simulink model "MODEL_FULL_SYSTEM_MUTUAL"  (Simulink 7.8)
settings: Solver=ode1  StartTime=0.0  StopTime=inf  FixedStep=Ts  MaxStep=1e-3  RelTol=1e-3
PostLoadFcn:
  | Ts=80e-6; relays_settings_init;
InitFcn:
  | Ts=80e-6; relays_settings_init;
values from neighbouring files (symbols this model uses):
  relay_sets = xlsread('relay_settings_10272015.xlsx')    [relays_settings_init.m]
undefined symbols (not defined in the file or in its folder): dfilt, DiscIntNeverNeededParam, fdesignblkfcn, gcbh, Left, opmodbus_cb, ph, Right, type, V, X
libraries: simulink x72, modbus_lib x40, cables_lib x36, rtio_opalrt_common x21, rtlab x20, transformer_lib x13, dynamic_load_lib x12, powerlib x6, simulink_extras x6, ssn_lib x5, discretizing x4, rteventslib x4
(part 5 of 7)

== system MODEL_FULL_SYSTEM_MUTUAL/SS_Slave/Input to UDP Block - v1 ==
  note: Using phase A:
      | 1)  voltage 1MVA gen
      | 2) voltage 4MVA gen
      | 3) battery current
  note: gens are operating at higher voltage than 1pu - instead of mult by 1.414, I mult by 1.214
  ms : Inport
  batt : Inport  Port=2
  gen : Inport  Port=3
  Bus Selector1 : BusSelector  OutputSignals=SEL_787_Relay1.m.P,SEL_787_Relay2.m.P,SEL_787_Relay3.m.P,SEL_787_Relay4.m.P,SEL_787_Relay5.m.P,SEL_787_Relay6.m.P,SEL_787_Relay7.m.P,SEL_787_Relay8.m.P,SEL_787_Relay9.m.P,SEL_787_Relay10.m.P,SEL_787_Relay11.m.P,SEL_787_Relay12.m.P,SEL_787_Relay13.m.P,SEL_787_Relay14.m.P,SEL_787_Relay15.m.P,SEL_787_Relay16.m.P,SEL_787_Relay17.m.P,SEL_787_Relay18.m.P,SEL_787_Relay19.m.P
  Bus Selector2 : BusSelector  OutputSignals=SEL_787_Relay1.m.Q,SEL_787_Relay2.m.Q,SEL_787_Relay3.m.Q,SEL_787_Relay4.m.Q,SEL_787_Relay5.m.Q,SEL_787_Relay6.m.Q,SEL_787_Relay7.m.Q,SEL_787_Relay8.m.Q,SEL_787_Relay9.m.Q,SEL_787_Relay10.m.Q,SEL_787_Relay11.m.Q,SEL_787_Relay12.m.Q,SEL_787_Relay13.m.Q,SEL_787_Relay14.m.Q,SEL_787_Relay15.m.Q,SEL_787_Relay16.m.Q,SEL_787_Relay17.m.Q,SEL_787_Relay18.m.Q,SEL_787_Relay19.m.Q
  Bus Selector3 : BusSelector  OutputSignals=SEL_787_Relay1.m.Vpu,SEL_787_Relay2.m.Vpu,SEL_787_Relay3.m.Vpu,SEL_787_Relay4.m.Vpu,SEL_787_Relay5.m.Vpu,SEL_787_Relay6.m.Vpu,SEL_787_Relay7.m.Vpu,SEL_787_Relay8.m.Vpu,SEL_787_Relay9.m.Vpu,SEL_787_Relay10.m.Vpu,SEL_787_Relay11.m.Vpu,SEL_787_Relay12.m.Vpu,SEL_787_Relay13.m.Vpu,SEL_787_Relay14.m.Vpu,SEL_787_Relay15.m.Vpu,SEL_787_Relay16.m.Vpu,SEL_787_Relay17.m.Vpu,SEL_787_Relay18.m.Vpu,SEL_787_Relay19.m.Vpu
  Bus Selector4 : BusSelector  OutputSignals=SEL_787_Relay1.m.freq,SEL_787_Relay2.m.freq,SEL_787_Relay3.m.freq,SEL_787_Relay4.m.freq,SEL_787_Relay5.m.freq,SEL_787_Relay6.m.freq,SEL_787_Relay7.m.freq,SEL_787_Relay8.m.freq,SEL_787_Relay9.m.freq,SEL_787_Relay10.m.freq,SEL_787_Relay11.m.freq,SEL_787_Relay12.m.freq,SEL_787_Relay13.m.freq,SEL_787_Relay14.m.freq,SEL_787_Relay15.m.freq,SEL_787_Relay16.m.freq,SEL_787_Relay17.m.freq,SEL_787_Relay18.m.freq,SEL_787_Relay19.m.freq
  Bus Selector5 : BusSelector  OutputSignals=SEL_787_Relay1.m.status,SEL_787_Relay2.m.status,SEL_787_Relay3.m.status,SEL_787_Relay4.m.status,SEL_787_Relay5.m.status,SEL_787_Relay6.m.status,SEL_787_Relay7.m.status,SEL_787_Relay8.m.status,SEL_787_Relay9.m.status,SEL_787_Relay10.m.status,SEL_787_Relay11.m.status,SEL_787_Relay12.m.status,SEL_787_Relay13.m.status,SEL_787_Relay14.m.status,SEL_787_Relay15.m.status,SEL_787_Relay16.m.status,SEL_787_Relay17.m.status,SEL_787_Relay18.m.status,SEL_787_Relay19.m.status
  Bus Selector6 : BusSelector  OutputSignals=Capacity.Capacity (signal 2)
  Bus Selector7 : BusSelector  OutputSignals=SEL_787_Relay1.m.pf
  Bus Selector8 : BusSelector  OutputSignals=gal_per_hr_1MVA,gal_per_hr_4MVA
  Bus Selector9 : BusSelector  OutputSignals=SEL_787_Relay7.m.Vabc,SEL_787_Relay8.m.Vabc,SEL_787_Relay13.m.Iabc
  Data Type Conversion : DataTypeConversion
  Demux : Demux  Outputs=3
  Demux1 : Demux  Outputs=3
  Demux2 : Demux  Outputs=3
  Gain : Gain  Gain=1.214/460
  Gain1 : Gain  Gain=1.214/13800
  Gain2 : Gain  Gain=1/1000
  Gain3 : Gain  Gain=1/1000
  Gain4 : Gain  Gain=1/(4E6/(1.732*2047))
  Mux : Mux  Inputs=3
  Mux{1..5} (5 alike) : Mux  Inputs=20
  Mux6 : Mux  Inputs=2
  waveforms : Outport
  kW : Outport  Port=2
  kvar : Outport  Port=3
  Vpu : Outport  Port=4
  freq : Outport  Port=5
  breaker_status : Outport  Port=6
  Batt SoC : Outport  Port=7
  PF at PCC : Outport  Port=8
  gen_fuel : Outport  Port=9
  wires:
  Bus Selector4/19 -> Mux4/19  "<freq>"
  Bus Selector4/18 -> Mux4/18  "<freq>"
  Bus Selector4/17 -> Mux4/17  "<freq>"
  Bus Selector4/16 -> Mux4/16  "<freq>"
  Bus Selector4/15 -> Mux4/15  "<freq>"
  Bus Selector4/14 -> Mux4/14  "<freq>"
  Bus Selector4/13 -> Mux4/13  "<freq>"
  Bus Selector4/12 -> Mux4/12  "<freq>"
  Bus Selector4/11 -> Mux4/11  "<freq>"
  Bus Selector4/10 -> Mux4/10  "<freq>"
  Bus Selector4/9 -> Mux4/9  "<freq>"
  Bus Selector4/8 -> Mux4/8  "<freq>"
  Bus Selector4/7 -> Mux4/7  "<freq>"
  Bus Selector4/6 -> Mux4/6  "<freq>"
  Bus Selector4/5 -> Mux4/5  "<freq>"
  Bus Selector4/4 -> Mux4/4  "<freq>"
  Bus Selector4/3 -> Mux4/3  "<freq>"
  Bus Selector4/2 -> Mux4/2  "<freq>"
  Bus Selector4/1 -> Mux4/1  "<freq>"
  Gain4/1 -> Demux2/1
  Data Type Conversion/1 -> breaker_status/1
  Bus Selector9/1 -> Gain/1  "<Vabc>"
  Bus Selector9/3 -> Gain4/1  "<Iabc>"
  Bus Selector9/2 -> Gain1/1  "<Vabc>"
  Demux1/1 -> Mux/2
  Demux/1 -> Mux/1
  Demux2/1 -> Mux/3
  Gain/1 -> Demux/1
  Gain1/1 -> Demux1/1
  ms/1 -> Bus Selector9/1, Bus Selector1/1, Bus Selector2/1, Bus Selector3/1, Bus Selector4/1, Bus Selector5/1, Bus Selector7/1
  Mux/1 -> waveforms/1
  Bus Selector1/1 -> Mux1/1  "<P>"
  Bus Selector1/2 -> Mux1/2  "<P>"
  Bus Selector1/3 -> Mux1/3  "<P>"
  Bus Selector1/4 -> Mux1/4  "<P>"
  Bus Selector1/5 -> Mux1/5  "<P>"
  Bus Selector1/6 -> Mux1/6  "<P>"
  Bus Selector1/7 -> Mux1/7  "<P>"
  Bus Selector1/8 -> Mux1/8  "<P>"
  Bus Selector1/9 -> Mux1/9  "<P>"
  Bus Selector1/10 -> Mux1/10  "<P>"
  Bus Selector1/11 -> Mux1/11  "<P>"
  Bus Selector1/12 -> Mux1/12  "<P>"
  Bus Selector1/13 -> Mux1/13  "<P>"
  Bus Selector1/14 -> Mux1/14  "<P>"
  Bus Selector1/15 -> Mux1/15  "<P>"
  Bus Selector1/16 -> Mux1/16  "<P>"
  Bus Selector1/17 -> Mux1/17  "<P>"
  Bus Selector1/18 -> Mux1/18  "<P>"
  Bus Selector1/19 -> Mux1/19  "<P>"
  Mux1/1 -> Gain2/1
  Gain2/1 -> kW/1
  Bus Selector2/1 -> Mux2/1  "<Q>"
  Bus Selector2/2 -> Mux2/2  "<Q>"
  Bus Selector2/3 -> Mux2/3  "<Q>"
  Bus Selector2/4 -> Mux2/4  "<Q>"
  Bus Selector2/5 -> Mux2/5  "<Q>"
  Bus Selector2/6 -> Mux2/6  "<Q>"
  Bus Selector2/7 -> Mux2/7  "<Q>"
  Bus Selector2/8 -> Mux2/8  "<Q>"
  Bus Selector2/9 -> Mux2/9  "<Q>"
  Bus Selector2/10 -> Mux2/10  "<Q>"
  Bus Selector2/11 -> Mux2/11  "<Q>"
  Bus Selector2/12 -> Mux2/12  "<Q>"
  Bus Selector2/13 -> Mux2/13  "<Q>"
  Bus Selector2/14 -> Mux2/14  "<Q>"
  Bus Selector2/15 -> Mux2/15  "<Q>"
  Bus Selector2/16 -> Mux2/16  "<Q>"
  Bus Selector2/17 -> Mux2/17  "<Q>"
  Bus Selector2/18 -> Mux2/18  "<Q>"
  Bus Selector2/19 -> Mux2/19  "<Q>"
  Mux2/1 -> Gain3/1
  Gain3/1 -> kvar/1
  Bus Selector3/1 -> Mux3/1  "<Vpu>"
  Bus Selector3/2 -> Mux3/2  "<Vpu>"
  Bus Selector3/3 -> Mux3/3  "<Vpu>"
  Bus Selector3/4 -> Mux3/4  "<Vpu>"
  Bus Selector3/5 -> Mux3/5  "<Vpu>"
  Bus Selector3/6 -> Mux3/6  "<Vpu>"
  Bus Selector3/7 -> Mux3/7  "<Vpu>"
  Bus Selector3/8 -> Mux3/8  "<Vpu>"
  Bus Selector3/9 -> Mux3/9  "<Vpu>"
  Bus Selector3/10 -> Mux3/10  "<Vpu>"
  Bus Selector3/11 -> Mux3/11  "<Vpu>"
  Bus Selector3/12 -> Mux3/12  "<Vpu>"
  Bus Selector3/13 -> Mux3/13  "<Vpu>"
  Bus Selector3/14 -> Mux3/14  "<Vpu>"
  Bus Selector3/15 -> Mux3/15  "<Vpu>"
  Bus Selector3/16 -> Mux3/16  "<Vpu>"
  Bus Selector3/17 -> Mux3/17  "<Vpu>"
  Bus Selector3/18 -> Mux3/18  "<Vpu>"
  Bus Selector3/19 -> Mux3/19  "<Vpu>"
  Mux3/1 -> Vpu/1
  Mux4/1 -> freq/1
  Mux5/1 -> Data Type Conversion/1
  batt/1 -> Bus Selector6/1
  Bus Selector6/1 -> Batt SoC/1  "<Capacity (signal 2)>"
  Bus Selector7/1 -> PF at PCC/1  "<pf>"
  Bus Selector5/1 -> Mux5/1  "<status>"
  Bus Selector5/2 -> Mux5/2  "<status>"
  Bus Selector5/3 -> Mux5/3  "<status>"
  Bus Selector5/4 -> Mux5/4  "<status>"
  Bus Selector5/5 -> Mux5/5  "<status>"
  Bus Selector5/6 -> Mux5/6  "<status>"
  Bus Selector5/7 -> Mux5/7  "<status>"
  Bus Selector5/8 -> Mux5/8  "<status>"
  Bus Selector5/9 -> Mux5/9  "<status>"
  Bus Selector5/10 -> Mux5/10  "<status>"
  Bus Selector5/11 -> Mux5/11  "<status>"
  Bus Selector5/12 -> Mux5/12  "<status>"
  Bus Selector5/13 -> Mux5/13  "<status>"
  Bus Selector5/14 -> Mux5/14  "<status>"
  Bus Selector5/15 -> Mux5/15  "<status>"
  Bus Selector5/16 -> Mux5/16  "<status>"
  Bus Selector5/17 -> Mux5/17  "<status>"
  Bus Selector5/18 -> Mux5/18  "<status>"
  Bus Selector5/19 -> Mux5/19  "<status>"
  gen/1 -> Bus Selector8/1
  Bus Selector8/1 -> Mux6/1  "<gal_per_hr_1MVA>"
  Bus Selector8/2 -> Mux6/2  "<gal_per_hr_4MVA>"
  Mux6/1 -> gen_fuel/1

== system MODEL_FULL_SYSTEM_MUTUAL/SS_Slave/Number of seconds of recording ==
  Compare To Constant1 : simulink/Logic and Bit Operations/Compare To Constant  relop=>=  const=time_s  OutDataTypeStr=boolean
  Increment : Subsystem
  Integrator : Integrator  ExternalReset=rising
  Memory : Memory
  Slope : Constant
  file suffix : Outport
  wires:
  Slope/1 -> Integrator/1
  Integrator/1 -> Compare To Constant1/1
  Compare To Constant1/1 -> Memory/1, Increment/Trigger  "limit reached"
  Memory/1 -> Integrator/2
  Increment/1(Out1) -> file suffix/1

== system MODEL_FULL_SYSTEM_MUTUAL/SS_Slave/Trigg_machine ==
  Write : Inport
  Odd : Inport  Port=2
  Even : Inport  Port=3
  Bitwise Operator : simulink/Logic and Bit Operations/Bitwise Operator  logicop=AND  UseBitMask=off  NumInputPorts=2  BitMask=bin2dec('11011001')  BitMaskRealWorld=Stored Integer
  Bitwise Operator1 : simulink/Logic and Bit Operations/Bitwise Operator  logicop=AND  UseBitMask=off  NumInputPorts=2  BitMask=bin2dec('11011001')  BitMaskRealWorld=Stored Integer
  Data Type Conversion : DataTypeConversion
  Data Type Conversion1 : DataTypeConversion
  Double2uint8 : DataTypeConversion
  Trig_odd : Outport
  Trig_even : Outport  Port=2
  wires:
  Double2uint8/1 -> Bitwise Operator1/1, Bitwise Operator/2
  Write/1 -> Double2uint8/1
  Odd/1 -> Bitwise Operator/1
  Data Type Conversion1/1 -> Trig_even/1
  Data Type Conversion/1 -> Trig_odd/1
  Even/1 -> Bitwise Operator1/2
  Bitwise Operator1/1 -> Data Type Conversion1/1
  Bitwise Operator/1 -> Data Type Conversion/1

== system MODEL_FULL_SYSTEM_MUTUAL/SS_Slave/isOddOrEven ==
  note: Si cette différence est égale à 0, c'est que le
      | nombre en entrée est pair, sinon c'est qu'il est impair.
  note: Effectuer la différence entre le nombre en entrée,
      | et sa moitié arrondie multipliée par 2.
  Index : Inport
  Compare To Zero : simulink/Logic and Bit Operations/Compare To Zero  relop=~=  OutDataTypeStr=boolean  ZeroCross=off
  Compare To Zero1 : simulink/Logic and Bit Operations/Compare To Zero  relop===  OutDataTypeStr=boolean  ZeroCross=off
  Constant3 : Constant  Value=2
  Divide : Product  Inputs=*/  OutDataTypeStr=double
  Produit : Product  Inputs=**  OutDataTypeStr=double
  Rounding Function : Rounding
  Sum : Sum  Inputs=|+-
  isOdd : Outport
  isEven : Outport  Port=2
  wires:
  Compare To Zero1/1 -> isEven/1
  Compare To Zero/1 -> isOdd/1
  Sum/1 -> Compare To Zero1/1, Compare To Zero/1
  Produit/1 -> Sum/2
  Rounding Function/1 -> Produit/1
  Index/1 -> Sum/1, Divide/1
  Divide/1 -> Rounding Function/1
  Constant3/1 -> Produit/2, Divide/2

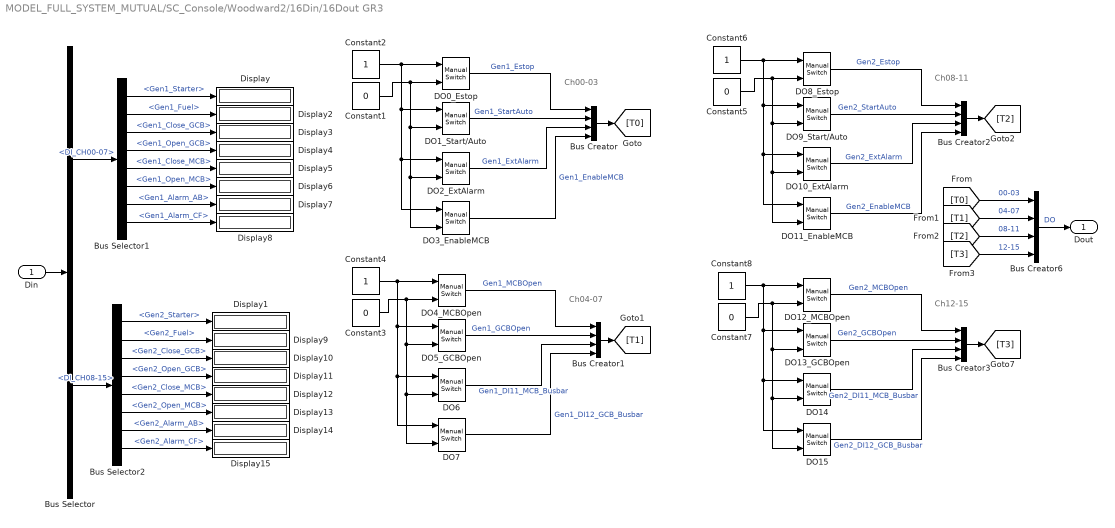
== system MODEL_FULL_SYSTEM_MUTUAL/SC_Console/Woodward2/16Din/16Dout GR3 ==
  note: Ch00-03
  note: Ch04-07
  note: Ch08-11
  note: Ch12-15
  Din : Inport
  Bus Creator{,1..3,6} (5 alike) : BusCreator
  Bus Selector : BusSelector  OutputSignals=DIN.DI_CH00-07,DIN.DI_CH08-15
  Bus Selector1 : BusSelector  OutputSignals=Gen1_Starter,Gen1_Fuel,Gen1_Close_GCB,Gen1_Open_GCB,Gen1_Close_MCB,Gen1_Open_MCB,Gen1_Alarm_AB,Gen1_Alarm_CF
  Bus Selector2 : BusSelector  OutputSignals=Gen2_Starter,Gen2_Fuel,Gen2_Close_GCB,Gen2_Open_GCB,Gen2_Close_MCB,Gen2_Open_MCB,Gen2_Alarm_AB,Gen2_Alarm_CF
  Constant{1,3,5,7} (4 alike) : Constant  Value=0
  Constant{2,4,6,8} (4 alike) : Constant
  DO0_Estop : simulink/Signal Routing/Manual Switch  sw=1  action=0  varsize=off
  DO10_ExtAlarm : simulink/Signal Routing/Manual Switch  sw=0  action=0  varsize=off
  DO11_EnableMCB : simulink/Signal Routing/Manual Switch  sw=0  action=0  varsize=off
  DO12_MCBOpen : simulink/Signal Routing/Manual Switch  sw=0  action=0  varsize=off
  DO13_GCBOpen : simulink/Signal Routing/Manual Switch  sw=0  action=0  varsize=off
  DO{6..7,14..15} (4 alike) : simulink/Signal Routing/Manual Switch  sw=0  action=0  varsize=off
  DO1_Start/Auto : simulink/Signal Routing/Manual Switch  sw=0  action=0  varsize=off
  DO2_ExtAlarm : simulink/Signal Routing/Manual Switch  sw=0  action=0  varsize=off
  DO3_EnableMCB : simulink/Signal Routing/Manual Switch  sw=0  action=0  varsize=off
  DO4_MCBOpen : simulink/Signal Routing/Manual Switch  sw=0  action=0  varsize=off
  DO5_GCBOpen : simulink/Signal Routing/Manual Switch  sw=0  action=0  varsize=off
  DO8_Estop : simulink/Signal Routing/Manual Switch  sw=1  action=0  varsize=off
  DO9_Start/Auto : simulink/Signal Routing/Manual Switch  sw=0  action=0  varsize=off
  Display{,1..15} (16 alike) : Display
  Dout : Outport
  wires:
  Bus Creator6/1 -> Dout/1  "DO"
  Constant2/1 -> DO0_Estop/1, DO1_Start/Auto/1, DO3_EnableMCB/1, DO2_ExtAlarm/1
  Constant1/1 -> DO0_Estop/2, DO1_Start/Auto/2, DO3_EnableMCB/2, DO2_ExtAlarm/2
  DO0_Estop/1 -> Bus Creator/1  "Gen1_Estop"
  DO1_Start/Auto/1 -> Bus Creator/2  "Gen1_StartAuto"
  DO2_ExtAlarm/1 -> Bus Creator/3  "Gen1_ExtAlarm"
  DO3_EnableMCB/1 -> Bus Creator/4  "Gen1_EnableMCB"
  Constant4/1 -> DO6/1, DO7/1, DO5_GCBOpen/1, DO4_MCBOpen/1
  Constant3/1 -> DO6/2, DO7/2, DO5_GCBOpen/2, DO4_MCBOpen/2
  DO4_MCBOpen/1 -> Bus Creator1/1  "Gen1_MCBOpen"
  DO5_GCBOpen/1 -> Bus Creator1/2  "Gen1_GCBOpen"
  DO6/1 -> Bus Creator1/3  "Gen1_DI11_MCB_Busbar"
  DO7/1 -> Bus Creator1/4  "Gen1_DI12_GCB_Busbar"
  Constant6/1 -> DO8_Estop/1, DO9_Start/Auto/1, DO11_EnableMCB/1, DO10_ExtAlarm/1
  Constant5/1 -> DO8_Estop/2, DO9_Start/Auto/2, DO11_EnableMCB/2, DO10_ExtAlarm/2
  DO8_Estop/1 -> Bus Creator2/1  "Gen2_Estop"
  DO9_Start/Auto/1 -> Bus Creator2/2  "Gen2_StartAuto"
  DO10_ExtAlarm/1 -> Bus Creator2/3  "Gen2_ExtAlarm"
  DO11_EnableMCB/1 -> Bus Creator2/4  "Gen2_EnableMCB"
  Constant8/1 -> DO14/1, DO15/1, DO13_GCBOpen/1, DO12_MCBOpen/1
  Constant7/1 -> DO14/2, DO15/2, DO13_GCBOpen/2, DO12_MCBOpen/2
  DO12_MCBOpen/1 -> Bus Creator3/1  "Gen2_MCBOpen"
  DO13_GCBOpen/1 -> Bus Creator3/2  "Gen2_GCBOpen"
  DO14/1 -> Bus Creator3/3  "Gen2_DI11_MCB_Busbar"
  DO15/1 -> Bus Creator3/4  "Gen2_DI12_GCB_Busbar"
  Bus Creator/1 -> [T0]
  Bus Creator1/1 -> [T1]
  Bus Creator3/1 -> [T3]
  Bus Creator2/1 -> [T2]
  [T0] -> Bus Creator6/1  "00-03"
  [T1] -> Bus Creator6/2  "04-07"
  [T2] -> Bus Creator6/3  "08-11"
  [T3] -> Bus Creator6/4  "12-15"
  Din/1 -> Bus Selector/1
  Bus Selector/1 -> Bus Selector1/1  "<DI_CH00-07>"
  Bus Selector1/1 -> Display/1  "<Gen1_Starter>"
  Bus Selector1/2 -> Display2/1  "<Gen1_Fuel>"
  Bus Selector1/3 -> Display3/1  "<Gen1_Close_GCB>"
  Bus Selector1/5 -> Display5/1  "<Gen1_Close_MCB>"
  Bus Selector1/6 -> Display6/1  "<Gen1_Open_MCB>"
  Bus Selector1/8 -> Display8/1  "<Gen1_Alarm_CF>"
  Bus Selector/2 -> Bus Selector2/1  "<DI_CH08-15>"
  Bus Selector2/1 -> Display1/1  "<Gen2_Starter>"
  Bus Selector2/2 -> Display9/1  "<Gen2_Fuel>"
  Bus Selector2/3 -> Display10/1  "<Gen2_Close_GCB>"
  Bus Selector2/4 -> Display11/1  "<Gen2_Open_GCB>"
  Bus Selector2/5 -> Display12/1  "<Gen2_Close_MCB>"
  Bus Selector2/6 -> Display13/1  "<Gen2_Open_MCB>"
  Bus Selector2/7 -> Display14/1  "<Gen2_Alarm_AB>"
  Bus Selector2/8 -> Display15/1  "<Gen2_Alarm_CF>"
  Bus Selector1/4 -> Display4/1  "<Gen1_Open_GCB>"
  Bus Selector1/7 -> Display7/1  "<Gen1_Alarm_AB>"

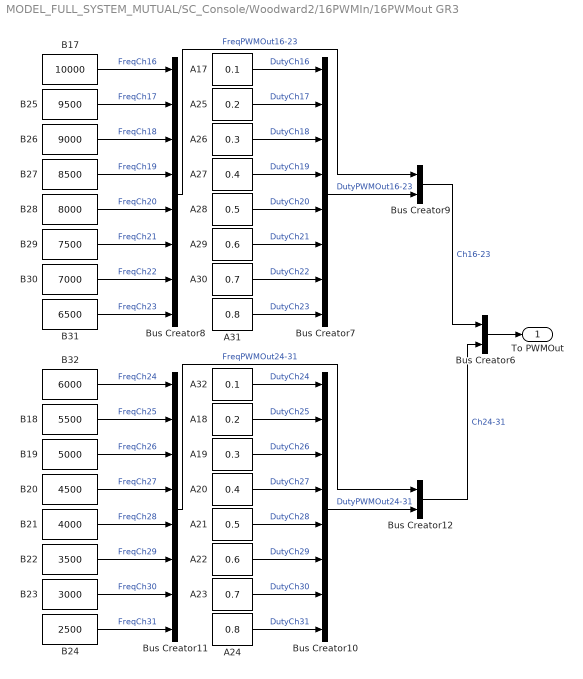
== system MODEL_FULL_SYSTEM_MUTUAL/SC_Console/Woodward2/16PWMIn/16PWMout GR3 ==
  A17 : Constant  Value=0.1
  A18 : Constant  Value=0.2
  A19 : Constant  Value=0.3
  A20 : Constant  Value=0.4
  A21 : Constant  Value=0.5
  A22 : Constant  Value=0.6
  A23 : Constant  Value=0.7
  A24 : Constant  Value=0.8
  A25 : Constant  Value=0.2
  A26 : Constant  Value=0.3
  A27 : Constant  Value=0.4
  A28 : Constant  Value=0.5
  A29 : Constant  Value=0.6
  A30 : Constant  Value=0.7
  A31 : Constant  Value=0.8
  A32 : Constant  Value=0.1
  B17 : Constant  Value=10000
  B18 : Constant  Value=5500
  B19 : Constant  Value=5000
  B20 : Constant  Value=4500
  B21 : Constant  Value=4000
  B22 : Constant  Value=3500
  B23 : Constant  Value=3000
  B24 : Constant  Value=2500
  B25 : Constant  Value=9500
  B26 : Constant  Value=9000
  B27 : Constant  Value=8500
  B28 : Constant  Value=8000
  B29 : Constant  Value=7500
  B30 : Constant  Value=7000
  B31 : Constant  Value=6500
  B32 : Constant  Value=6000
  Bus Creator{7..8,10..11} (4 alike) : BusCreator  Inputs=8
  Bus Creator12 : BusCreator  Inputs=2
  Bus Creator6 : BusCreator  Inputs=2
  Bus Creator9 : BusCreator  Inputs=2
  To PWMOut : Outport
  wires:
  Bus Creator6/1 -> To PWMOut/1
  A17/1 -> Bus Creator7/1  "DutyCh16"
  A25/1 -> Bus Creator7/2  "DutyCh17"
  A26/1 -> Bus Creator7/3  "DutyCh18"
  A27/1 -> Bus Creator7/4  "DutyCh19"
  A28/1 -> Bus Creator7/5  "DutyCh20"
  A29/1 -> Bus Creator7/6  "DutyCh21"
  A30/1 -> Bus Creator7/7  "DutyCh22"
  A31/1 -> Bus Creator7/8  "DutyCh23"
  B17/1 -> Bus Creator8/1  "FreqCh16"
  B25/1 -> Bus Creator8/2  "FreqCh17"
  B26/1 -> Bus Creator8/3  "FreqCh18"
  B27/1 -> Bus Creator8/4  "FreqCh19"
  B28/1 -> Bus Creator8/5  "FreqCh20"
  B29/1 -> Bus Creator8/6  "FreqCh21"
  B30/1 -> Bus Creator8/7  "FreqCh22"
  B31/1 -> Bus Creator8/8  "FreqCh23"
  Bus Creator7/1 -> Bus Creator9/2  "DutyPWMOut16-23"
  Bus Creator8/1 -> Bus Creator9/1  "FreqPWMOut16-23"
  A32/1 -> Bus Creator10/1  "DutyCh24"
  A18/1 -> Bus Creator10/2  "DutyCh25"
  A19/1 -> Bus Creator10/3  "DutyCh26"
  A20/1 -> Bus Creator10/4  "DutyCh27"
  A21/1 -> Bus Creator10/5  "DutyCh28"
  A22/1 -> Bus Creator10/6  "DutyCh29"
  A23/1 -> Bus Creator10/7  "DutyCh30"
  A24/1 -> Bus Creator10/8  "DutyCh31"
  B32/1 -> Bus Creator11/1  "FreqCh24"
  B18/1 -> Bus Creator11/2  "FreqCh25"
  B19/1 -> Bus Creator11/3  "FreqCh26"
  B20/1 -> Bus Creator11/4  "FreqCh27"
  B21/1 -> Bus Creator11/5  "FreqCh28"
  B22/1 -> Bus Creator11/6  "FreqCh29"
  B23/1 -> Bus Creator11/7  "FreqCh30"
  B24/1 -> Bus Creator11/8  "FreqCh31"
  Bus Creator10/1 -> Bus Creator12/2  "DutyPWMOut24-31"
  Bus Creator11/1 -> Bus Creator12/1  "FreqPWMOut24-31"
  Bus Creator12/1 -> Bus Creator6/2  "Ch24-31"
  Bus Creator9/1 -> Bus Creator6/1  "Ch16-23"

== system MODEL_FULL_SYSTEM_MUTUAL/SC_Console/Woodward2/16TSDIn/16 TSDOut GR3 ==
  Bus Creator1 : BusCreator  Inputs=3
  Din/Dout ch16-23 : Subsystem
  Din/Dout ch24-31 : Subsystem
  Dout state ctrl : Subsystem
  TSDout : Outport
  wires:
  Din/Dout ch24-31/1(Out1) -> Bus Creator1/2  "times CH24-31"
  Din/Dout ch16-23/1(Out1) -> Bus Creator1/1  "times CH16-23"
  Dout state ctrl/1(Event State OUT) -> Bus Creator1/3  "states"
  Bus Creator1/1 -> TSDout/1

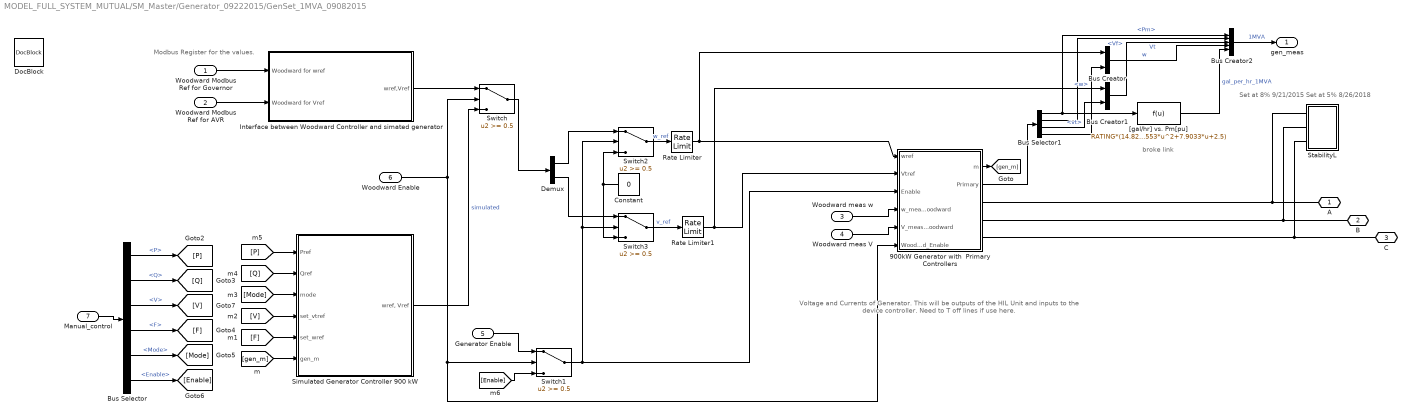
== system MODEL_FULL_SYSTEM_MUTUAL/SM_Master/Generator_09222015/GenSet_1MVA_09082015 ==
  note: Modbus Register for the values.
  note: Voltage and Currents of Generator.
      | This will be outputs of the HIL Unit
      | and inputs to the device controller.
      | Need to T off lines if use here.
  note: Set at 8% 9/21/2015
      | Set at 5% 8/26/2018
  note: broke link
  Woodward Modbus Ref for Governor : Inport
  Woodward Modbus Ref for AVR : Inport  Port=2
  Woodward meas w : Inport  Port=3
  Woodward meas V : Inport  Port=4
  Generator Enable : Inport  Port=5
  Woodward Enable : Inport  Port=6
  Manual_control : Inport  Port=7
  900kW Generator with  Primary Controllers : Subsystem
  Bus Creator : BusCreator  Inputs=2
  Bus Creator1 : BusCreator  Inputs=2
  Bus Creator2 : BusCreator  Inputs=5
  Bus Selector : BusSelector  OutputSignals=P,Q,V,F,Mode,Enable
  Bus Selector1 : BusSelector  OutputSignals=Pm,Vf,vt,w
  Constant : Constant  Value=0
  Demux : Demux  Outputs=2
  DocBlock : simulink/Model-Wide Utilities/DocBlock  DocumentType=Text
  Interface between Woodward Controller and simated generator : Subsystem
  Rate Limiter : RateLimiter  RisingSlewLimit=0.5  FallingSlewLimit=-0.5  SampleTimeMode=inherited
  Rate Limiter1 : RateLimiter  RisingSlewLimit=0.5  FallingSlewLimit=-0.5  SampleTimeMode=inherited
  Simulated Generator Controller 900 kW : Subsystem
  StabilityL : Subsystem  mask{v=460, kVA=80, pf=1}
  Switch{,1..3} (4 alike) : Switch  Threshold=0.5
  "[gal/hr] vs. Pm[pu]" : Fcn  Expr=RATING*(14.827*u^4-27.253*u^3+15.553*u^2+7.9033*u+2.5)  mask{RATING=1}
      mask prompts: RATING "Rating [MW]"
      mask help: This block computes the gal/hr vs Pm[pu] of a generator of a given rating [MW].
  A : PMIOPort  Port=1  Side=Right
  B : PMIOPort  Port=2  Side=Right
  C : PMIOPort  Port=3  Side=Right
  gen_meas : Outport
  wires:
  [F] -> Simulated Generator Controller 900 kW/5(set_wref)
  [V] -> Simulated Generator Controller 900 kW/4(set_vtref)
  [Mode] -> Simulated Generator Controller 900 kW/3(mode)
  [Q] -> Simulated Generator Controller 900 kW/2(Qref)
  [P] -> Simulated Generator Controller 900 kW/1(Pref)
  [gen_m] -> Simulated Generator Controller 900 kW/6(gen_m)
  Bus Selector/5 -> [Mode]  "<Mode>"
  Bus Selector/4 -> [F]  "<F>"
  Bus Selector/3 -> [V]  "<V>"
  Bus Selector/2 -> [Q]  "<Q>"
  Bus Selector/1 -> [P]  "<P>"
  Manual_control/1 -> Bus Selector/1
  Simulated Generator Controller 900 kW/1("wref, Vref") -> Switch/3  "simulated"
  900kW Generator with  Primary Controllers/1(m) -> [gen_m]
  Interface between Woodward Controller and simated generator/1(wref,Vref) -> Switch/1
  Switch/1 -> Demux/1
  Woodward Modbus Ref for Governor/1 -> Interface between Woodward Controller and simated generator/1(Woodward for wref)
  Woodward Modbus Ref for AVR/1 -> Interface between Woodward Controller and simated generator/2(Woodward for Vref)
  Woodward meas w/1 -> 900kW Generator with  Primary Controllers/4(w_meas_Woodward)
  Woodward meas V/1 -> 900kW Generator with  Primary Controllers/5(V_meas_Woodward)
  Bus Selector/6 -> [Enable]  "<Enable>"
  900kW Generator with  Primary Controllers/2(Primary) -> Bus Selector1/1
  Generator Enable/1 -> Switch1/1
  [Enable] -> Switch1/3
  Switch1/1 -> 900kW Generator with  Primary Controllers/3(Enable), Switch2/2, Switch3/2
  Switch2/1 -> Rate Limiter/1  "w_ref"
  Demux/1 -> Switch2/1
  Demux/2 -> Switch3/1
  Constant/1 -> Switch3/3, Switch2/3
  Switch3/1 -> Rate Limiter1/1  "v_ref"
  Bus Selector1/3 -> Bus Creator1/2  "<vt>"
  Bus Selector1/4 -> Bus Creator/2  "<w>"
  Bus Selector1/2 -> Bus Creator2/2  "<Vf>"
  Bus Selector1/1 -> Bus Creator2/1, "[gal/hr] vs. Pm[pu]"/1  "<Pm>"
  Bus Creator1/1 -> Bus Creator2/3  "Vt"
  Bus Creator/1 -> Bus Creator2/4  "w"
  Bus Creator2/1 -> gen_meas/1  "1MVA"
  Rate Limiter/1 -> 900kW Generator with  Primary Controllers/1(wref), Bus Creator/1
  Rate Limiter1/1 -> 900kW Generator with  Primary Controllers/2(Vtref), Bus Creator1/1
  Woodward Enable/1 -> Switch/2, Switch1/2, 900kW Generator with  Primary Controllers/6(Woodward_Enable)
  "[gal/hr] vs. Pm[pu]"/1 -> Bus Creator2/5  "gal_per_hr_1MVA"
  connections:
  900kW Generator with  Primary Controllers/RConn3 -- StabilityL/LConn3 -- C/RConn1
  900kW Generator with  Primary Controllers/RConn2 -- StabilityL/LConn2 -- B/RConn1
  900kW Generator with  Primary Controllers/RConn1 -- StabilityL/LConn1 -- A/RConn1

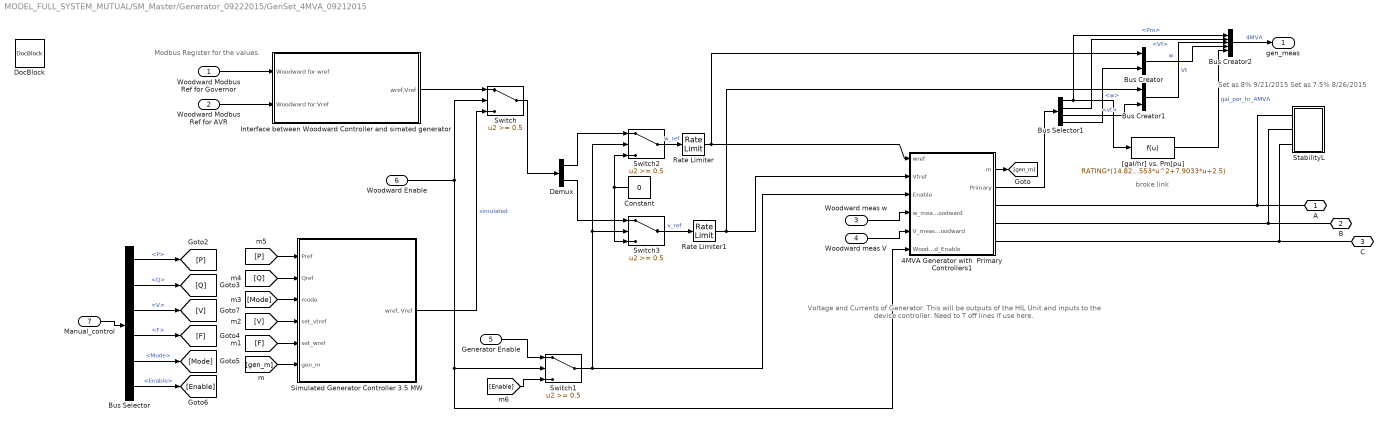
== system MODEL_FULL_SYSTEM_MUTUAL/SM_Master/Generator_09222015/GenSet_4MVA_09212015 ==
  note: Modbus Register for the values.
  note: Voltage and Currents of Generator.
      | This will be outputs of the HIL Unit
      | and inputs to the device controller.
      | Need to T off lines if use here.
  note: Set as 8% 9/21/2015
      | Set as 7.5% 8/26/2015
  note: broke link
  Woodward Modbus Ref for Governor : Inport
  Woodward Modbus Ref for AVR : Inport  Port=2
  Woodward meas w : Inport  Port=3
  Woodward meas V : Inport  Port=4
  Generator Enable : Inport  Port=5
  Woodward Enable : Inport  Port=6
  Manual_control : Inport  Port=7
  4MVA Generator with  Primary Controllers1 : Subsystem
  Bus Creator : BusCreator  Inputs=2
  Bus Creator1 : BusCreator  Inputs=2
  Bus Creator2 : BusCreator  Inputs=5
  Bus Selector : BusSelector  OutputSignals=P,Q,V,F,Mode,Enable
  Bus Selector1 : BusSelector  OutputSignals=Pm,Vf,vt,w
  Constant : Constant  Value=0
  Demux : Demux  Outputs=2
  DocBlock : simulink/Model-Wide Utilities/DocBlock  DocumentType=Text
  Interface between Woodward Controller and simated generator : Subsystem
  Rate Limiter : RateLimiter  RisingSlewLimit=0.5  FallingSlewLimit=-0.5  SampleTimeMode=inherited
  Rate Limiter1 : RateLimiter  RisingSlewLimit=0.5  FallingSlewLimit=-0.5  SampleTimeMode=inherited
  Simulated Generator Controller 3.5 MW : Subsystem
  StabilityL : Subsystem  mask{v=13800, kVA=320, pf=1}
  Switch{,1..3} (4 alike) : Switch  Threshold=0.5
  "[gal/hr] vs. Pm[pu]" : Fcn  Expr=RATING*(14.827*u^4-27.253*u^3+15.553*u^2+7.9033*u+2.5)  mask{RATING=4}
      mask prompts: RATING "Rating [MW]"
      mask help: This block computes the gal/hr vs Pm[pu] of a generator of a given rating [MW].
  A : PMIOPort  Port=1  Side=Right
  B : PMIOPort  Port=2  Side=Right
  C : PMIOPort  Port=3  Side=Right
  gen_meas : Outport
  wires:
  [F] -> Simulated Generator Controller 3.5 MW/5(set_wref)
  [V] -> Simulated Generator Controller 3.5 MW/4(set_vtref)
  [Mode] -> Simulated Generator Controller 3.5 MW/3(mode)
  [Q] -> Simulated Generator Controller 3.5 MW/2(Qref)
  [P] -> Simulated Generator Controller 3.5 MW/1(Pref)
  [gen_m] -> Simulated Generator Controller 3.5 MW/6(gen_m)
  Bus Selector/5 -> [Mode]  "<Mode>"
  Bus Selector/4 -> [F]  "<F>"
  Bus Selector/3 -> [V]  "<V>"
  Bus Selector/2 -> [Q]  "<Q>"
  Bus Selector/1 -> [P]  "<P>"
  Manual_control/1 -> Bus Selector/1
  Simulated Generator Controller 3.5 MW/1("wref, Vref") -> Switch/3  "simulated"
  4MVA Generator with  Primary Controllers1/1(m) -> [gen_m]
  Interface between Woodward Controller and simated generator/1(wref,Vref) -> Switch/1
  Switch/1 -> Demux/1
  Woodward Modbus Ref for Governor/1 -> Interface between Woodward Controller and simated generator/1(Woodward for wref)
  Woodward Modbus Ref for AVR/1 -> Interface between Woodward Controller and simated generator/2(Woodward for Vref)
  Woodward meas w/1 -> 4MVA Generator with  Primary Controllers1/4(w_meas_Woodward)
  Woodward meas V/1 -> 4MVA Generator with  Primary Controllers1/5(V_meas_Woodward)
  Bus Selector/6 -> [Enable]  "<Enable>"
  4MVA Generator with  Primary Controllers1/2(Primary) -> Bus Selector1/1
  Generator Enable/1 -> Switch1/1
  [Enable] -> Switch1/3
  Switch1/1 -> 4MVA Generator with  Primary Controllers1/3(Enable), Switch2/2, Switch3/2
  Switch2/1 -> Rate Limiter/1  "w_ref"
  Demux/1 -> Switch2/1
  Demux/2 -> Switch3/1
  Constant/1 -> Switch3/3, Switch2/3
  Switch3/1 -> Rate Limiter1/1  "v_ref"
  Bus Selector1/3 -> Bus Creator1/2  "<vt>"
  Bus Selector1/4 -> Bus Creator/2  "<w>"
  Bus Selector1/2 -> Bus Creator2/2  "<Vf>"
  Bus Selector1/1 -> Bus Creator2/1, "[gal/hr] vs. Pm[pu]"/1  "<Pm>"
  Bus Creator1/1 -> Bus Creator2/3  "Vt"
  Bus Creator/1 -> Bus Creator2/4  "w"
  Bus Creator2/1 -> gen_meas/1  "4MVA"
  Rate Limiter/1 -> 4MVA Generator with  Primary Controllers1/1(wref), Bus Creator/1
  Rate Limiter1/1 -> 4MVA Generator with  Primary Controllers1/2(Vtref), Bus Creator1/1
  Woodward Enable/1 -> Switch/2, 4MVA Generator with  Primary Controllers1/6(Woodward_Enable), Switch1/2
  "[gal/hr] vs. Pm[pu]"/1 -> Bus Creator2/5  "gal_per_hr_4MVA"
  connections:
  StabilityL/LConn1 -- A/RConn1 -- 4MVA Generator with  Primary Controllers1/RConn1
  StabilityL/LConn2 -- B/RConn1 -- 4MVA Generator with  Primary Controllers1/RConn2
  StabilityL/LConn3 -- C/RConn1 -- 4MVA Generator with  Primary Controllers1/RConn3

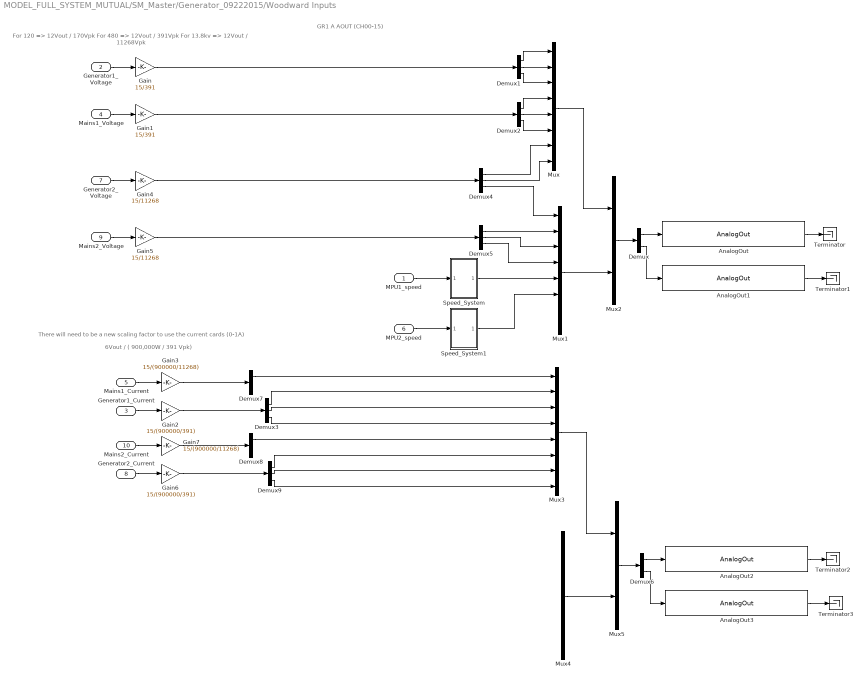
== system MODEL_FULL_SYSTEM_MUTUAL/SM_Master/Generator_09222015/Woodward Inputs ==
  note: 6Vout / ( 900,000W / 391 Vpk)
  note: For 120 => 12Vout / 170Vpk
      | For 480 => 12Vout / 391Vpk
      | For 13.8kv => 12Vout / 11268Vpk
  note: GR1 A AOUT (CH00-15)
  note: There will need to be a
      | new scaling factor to use
      | the current cards (0-1A)
  MPU1_speed : Inport
  Generator1_Voltage : Inport  Port=2
  Generator1_Current : Inport  Port=3
  Mains1_Voltage : Inport  Port=4
  Mains1_Current : Inport  Port=5
  MPU2_speed : Inport  Port=6
  Generator2_Voltage : Inport  Port=7
  Generator2_Current : Inport  Port=8
  Mains2_Voltage : Inport  Port=9
  Mains2_Current : Inport  Port=10
  AnalogOut : rtio_opalrt_common/AnalogOut  CtrlName='OpCtrl'  portNb=1  FcnNos=Slot 1 Module A Subsection 1  size=16  maxcount=8  count=8  numchan=8  israngeinput=off  voltagerange=[-16 ... 16]  slot=0  side=0  mismatch=0  slotside=Slot_1_Module_A
      settings: AttributesFormatString=%<CtrlName>
  AnalogOut1 : rtio_opalrt_common/AnalogOut  CtrlName='OpCtrl'  portNb=2  FcnNos=Slot 1 Module A Subsection 2  size=16  maxcount=8  count=8  numchan=8  israngeinput=off  voltagerange=[-16 ... 16]  slot=0  side=0  mismatch=0  slotside=Slot_1_Module_A
      settings: AttributesFormatString=%<CtrlName>
  AnalogOut2 : rtio_opalrt_common/AnalogOut  CtrlName='OpCtrl'  portNb=3  FcnNos=Slot 2 Module A Subsection 1  size=16  maxcount=8  count=8  numchan=8  israngeinput=off  voltagerange=[-16 ... 16]  slot=1  side=0  mismatch=0  slotside=Slot_2_Module_A
      settings: AttributesFormatString=%<CtrlName>
  AnalogOut3 : rtio_opalrt_common/AnalogOut  CtrlName='OpCtrl'  portNb=4  FcnNos=Slot 2 Module A Subsection 2  size=16  maxcount=8  count=8  numchan=8  israngeinput=off  voltagerange=[-16 ... 16]  slot=1  side=0  mismatch=0  slotside=Slot_2_Module_A
      settings: AttributesFormatString=%<CtrlName>
  Demux : Demux  Outputs=2
  Demux{1..5,7..9} (8 alike) : Demux  Outputs=3
  Demux6 : Demux  Outputs=2
  Gain : Gain  Gain=15/391
  Gain1 : Gain  Gain=15/391
  Gain2 : Gain  Gain=15/(900000/391)
  Gain3 : Gain  Gain=15/(900000/11268)
  Gain4 : Gain  Gain=15/11268
  Gain5 : Gain  Gain=15/11268
  Gain6 : Gain  Gain=15/(900000/391)
  Gain7 : Gain  Gain=15/(900000/11268)
  Mux{,1,3..4} (4 alike) : Mux  Inputs=8
  Mux2 : Mux  Inputs=2
  Mux5 : Mux  Inputs=2
  Speed_System : Subsystem
  Speed_System1 : Subsystem
  Terminator{,1..3} (4 alike) : Terminator
  wires:
  MPU1_speed/1 -> Speed_System/1(In1)
  Generator1_Current/1 -> Gain2/1
  Gain1/1 -> Demux2/1
  Gain/1 -> Demux1/1
  Mains1_Voltage/1 -> Gain1/1
  Mux2/1 -> Demux/1
  Mux1/1 -> Mux2/2
  Mux/1 -> Mux2/1
  Generator1_Voltage/1 -> Gain/1
  Demux/2 -> AnalogOut1/1
  Demux/1 -> AnalogOut/1
  AnalogOut1/1 -> Terminator1/1
  AnalogOut/1 -> Terminator/1
  Demux1/1 -> Mux/1
  Demux1/2 -> Mux/2
  Demux1/3 -> Mux/3
  Demux2/1 -> Mux/4
  Demux2/2 -> Mux/5
  Demux2/3 -> Mux/6
  Speed_System/1(Out1) -> Mux1/5
  Demux4/1 -> Mux/7
  Demux4/2 -> Mux/8
  Demux4/3 -> Mux1/1
  Demux5/1 -> Mux1/2
  Demux5/2 -> Mux1/3
  Demux5/3 -> Mux1/4
  Mux5/1 -> Demux6/1
  Mux4/1 -> Mux5/2
  Mux3/1 -> Mux5/1
  Demux6/2 -> AnalogOut3/1
  Demux6/1 -> AnalogOut2/1
  AnalogOut3/1 -> Terminator3/1
  AnalogOut2/1 -> Terminator2/1
  Gain2/1 -> Demux3/1
  Demux3/1 -> Mux3/2
  Demux3/2 -> Mux3/3
  Demux3/3 -> Mux3/4
  Mains1_Current/1 -> Gain3/1
  Gain3/1 -> Demux7/1
  Demux7/1 -> Mux3/1
  Gain5/1 -> Demux5/1
  Gain4/1 -> Demux4/1
  Mains2_Voltage/1 -> Gain5/1
  Generator2_Voltage/1 -> Gain4/1
  MPU2_speed/1 -> Speed_System1/1(In1)
  Speed_System1/1(Out1) -> Mux1/6
  Generator2_Current/1 -> Gain6/1
  Mains2_Current/1 -> Gain7/1
  Gain7/1 -> Demux8/1
  Demux8/1 -> Mux3/5
  Gain6/1 -> Demux9/1
  Demux9/1 -> Mux3/6
  Demux9/2 -> Mux3/7
  Demux9/3 -> Mux3/8

== system MODEL_FULL_SYSTEM_MUTUAL/SM_Master/Generator_09222015/Woodward Outputs ==
  Digital Output : Inport
  DIO Enable : Inport  Port=2
  Bias Enable : Inport  Port=3
  Gen1 MCB Status : Inport  Port=4
  Gen2 MCB Status : Inport  Port=5
  Bus Creator1 : BusCreator  Inputs=3
  DIO - Gr3 : Subsystem
  DIO - Woodward : Subsystem
  DOUT type config : Subsystem
  OpCtrl : rtio_opalrt_common/OpCtrl  CtrlName='OpCtrl'  boardid=0  BitstreamFilename=VC707_2-EX-0001-2_2_6_61-32AIO16DIO16DIOSel-01-01.bin  numconfig=-1  mode=Master  externalClock=off  decimRtsi=0  calibIO=off  SampleTime=0  loadinport=-1  BoardType=VC707  SecondaryPresent=off  sync_type=Audio
  PWM IO - Gr3 : Subsystem
  TSDIO - Gr3 : Subsystem
  Woodward Primary Inputs : Subsystem
  Error : Outport
  IDs : Outport  Port=2
  Digital Inputs : Outport  Port=3
  Gen1 Gov and AVR : Outport  Port=4
  Gen2 Gov and AVR : Outport  Port=5
  Gen1 Fuel Enable : Outport  Port=6
  Gen1 GCB : Outport  Port=7
  Gen1 MCB : Outport  Port=8
  Gen2 Fuel Enable : Outport  Port=9
  Gen2 GCB : Outport  Port=10
  Gen2 MCB : Outport  Port=11
  wires:
  OpCtrl/1 -> Error/1
  OpCtrl/2 -> IDs/1
  DIO - Woodward/4(DIn1) -> DIO - Gr3/1(Dout)
  PWM IO - Gr3/1(PWMIn) -> Bus Creator1/3  "PWMIN"
  TSDIO - Gr3/1(TSDin) -> Bus Creator1/2  "TSDIN"
  DIO - Gr3/1(DIn) -> Bus Creator1/1, DIO - Woodward/1(Din_Wood1)  "DIN"
  Bus Creator1/1 -> Digital Inputs/1
  DIO Enable/1 -> DIO - Woodward/3(control), DIO - Woodward/4(control1)
  Woodward Primary Inputs/1(Gen1 Gov and AVR) -> Gen1 Gov and AVR/1
  Woodward Primary Inputs/2(Gen2 Gov and AVR) -> Gen2 Gov and AVR/1
  Bias Enable/1 -> Woodward Primary Inputs/1(Bias-ctrl)
  Digital Output/1 -> DIO - Woodward/2(Din_sim), PWM IO - Gr3/1(PWMOut), TSDIO - Gr3/1(TSDout)
  DIO - Woodward/1(Gen1 Fuel Enable) -> Gen1 Fuel Enable/1
  DIO - Woodward/6(Gen2 GCB) -> Gen2 GCB/1
  DIO - Woodward/5(Gen2 Fuel Enable) -> Gen2 Fuel Enable/1
  DIO - Woodward/7(Gen2 MCB) -> Gen2 MCB/1
  Gen1 MCB Status/1 -> DIO - Woodward/5(Gen1 MCB Status)
  Gen2 MCB Status/1 -> DIO - Woodward/6(Gen2 MCB Status)
  DIO - Woodward/2(Gen1 GCB) -> Gen1 GCB/1
  DIO - Woodward/3(Gen1 MCB) -> Gen1 MCB/1

== system MODEL_FULL_SYSTEM_MUTUAL/SS_Slave/BATT_MODBUS/bitwise_faults ==
  note: Constant array has LSB on most left.
  batt_fault : Inport
  Bitwise Operator : simulink/Logic and Bit Operations/Bitwise Operator  logicop=OR  UseBitMask=off  NumInputPorts=8  BitMask=bin2dec('11011001')  BitMaskRealWorld=Stored Integer
  Data Type Conversion : DataTypeConversion  OutDataTypeStr=uint16
  Data Type Conversion1 : DataTypeConversion
  Demux : Demux  Outputs=8
  Shift Arithmetic : ArithShift  BitShiftNumber=1  BitShiftDirection=Left
  Shift Arithmetic1 : ArithShift  BitShiftNumber=2  BitShiftDirection=Left
  Shift Arithmetic2 : ArithShift  BitShiftNumber=3  BitShiftDirection=Left
  Shift Arithmetic3 : ArithShift  BitShiftNumber=4  BitShiftDirection=Left
  Shift Arithmetic4 : ArithShift  BitShiftNumber=5  BitShiftDirection=Left
  Shift Arithmetic5 : ArithShift  BitShiftNumber=6  BitShiftDirection=Left
  Shift Arithmetic6 : ArithShift  BitShiftNumber=7  BitShiftDirection=Left
  to_mb : Outport
  wires:
  Data Type Conversion1/1 -> to_mb/1
  Bitwise Operator/1 -> Data Type Conversion1/1
  batt_fault/1 -> Data Type Conversion/1
  Demux/6 -> Shift Arithmetic4/1
  Demux/5 -> Shift Arithmetic3/1
  Demux/4 -> Shift Arithmetic2/1
  Demux/3 -> Shift Arithmetic1/1
  Demux/2 -> Shift Arithmetic/1
  Demux/1 -> Bitwise Operator/1
  Data Type Conversion/1 -> Demux/1
  Demux/7 -> Shift Arithmetic5/1
  Demux/8 -> Shift Arithmetic6/1
  Shift Arithmetic/1 -> Bitwise Operator/2
  Shift Arithmetic1/1 -> Bitwise Operator/3
  Shift Arithmetic2/1 -> Bitwise Operator/4
  Shift Arithmetic3/1 -> Bitwise Operator/5
  Shift Arithmetic4/1 -> Bitwise Operator/6
  Shift Arithmetic5/1 -> Bitwise Operator/7
  Shift Arithmetic6/1 -> Bitwise Operator/8

== system MODEL_FULL_SYSTEM_MUTUAL/SS_Slave/Number of seconds of recording/Increment ==
  Trigger : TriggerPort
  Increment : Constant
  Memory : Memory  InheritSampleTime=on
  Sum : Sum  Inputs=|++
  Out1 : Outport
  wires:
  Sum/1 -> Out1/1, Memory/1
  Memory/1 -> Sum/1
  Increment/1 -> Sum/2

== system MODEL_FULL_SYSTEM_MUTUAL/SC_Console/Woodward2/16TSDIn/16 TSDOut GR3/Din/Dout ch16-23 ==
  Bus Creator3 : BusCreator  Inputs=8
  times17 : Constant  Value=[0.05 0.15 0.25 0.35]
  times18 : Constant  Value=[0.1 0.2 0.3 0.4]
  times19 : Constant  Value=[0.15 0.25 0.35 0.45]
  times20 : Constant  Value=[0.2 0.3 0.4 0.5]
  times21 : Constant  Value=[0.25 0.35 0.45 0.55]
  times22 : Constant  Value=[0.3 0.4 0.5 0.6]
  times23 : Constant  Value=[0.3 0.4 0.5 0.6]
  times24 : Constant  Value=[0 0.1 0.2 0.3]
  Out1 : Outport
  wires:
  Bus Creator3/1 -> Out1/1
  times23/1 -> Bus Creator3/8  "times24"
  times22/1 -> Bus Creator3/7  "times23"
  times21/1 -> Bus Creator3/6  "times22"
  times20/1 -> Bus Creator3/5  "times21"
  times19/1 -> Bus Creator3/4  "times20"
  times18/1 -> Bus Creator3/3  "times19"
  times17/1 -> Bus Creator3/2  "times18"
  times24/1 -> Bus Creator3/1  "times17"

== system MODEL_FULL_SYSTEM_MUTUAL/SC_Console/Woodward2/16TSDIn/16 TSDOut GR3/Din/Dout ch24-31 ==
  Bus Creator4 : BusCreator  Inputs=8
  times25 : Constant  Value=[0.05 0.15 0.25 0.35]
  times26 : Constant  Value=[0.1 0.2 0.3 0.4]
  times27 : Constant  Value=[0.15 0.25 0.35 0.45]
  times28 : Constant  Value=[0.2 0.3 0.4 0.5]
  times29 : Constant  Value=[0.25 0.35 0.45 0.55]
  times30 : Constant  Value=[0.3 0.4 0.5 0.6]
  times31 : Constant  Value=[0.3 0.4 0.5 0.6]
  times32 : Constant  Value=[0 0.1 0.2 0.3]
  Out1 : Outport
  wires:
  Bus Creator4/1 -> Out1/1
  times31/1 -> Bus Creator4/8  "times32"
  times30/1 -> Bus Creator4/7  "times31"
  times29/1 -> Bus Creator4/6  "times30"
  times28/1 -> Bus Creator4/5  "times29"
  times27/1 -> Bus Creator4/4  "times28"
  times26/1 -> Bus Creator4/3  "times27"
  times25/1 -> Bus Creator4/2  "times26"
  times32/1 -> Bus Creator4/1  "times25"

== system MODEL_FULL_SYSTEM_MUTUAL/SC_Console/Woodward2/16TSDIn/16 TSDOut GR3/Dout state ctrl ==
  Bus Creator : BusCreator  Inputs=2
  Dout_CH16_CH23 : Subsystem
  Dout_CH24_CH31 : Subsystem
  Event State OUT : Outport
  wires:
  Dout_CH24_CH31/1(Dout_CH8_CH15) -> Bus Creator/2  "CH24-31"
  Dout_CH16_CH23/1(Dout_CH8_CH15) -> Bus Creator/1  "CH16-23"
  Bus Creator/1 -> Event State OUT/1

== system MODEL_FULL_SYSTEM_MUTUAL/SM_Master/Generator_09222015/GenSet_1MVA_09082015/900kW Generator with  Primary Controllers ==
  wref : Inport
  Vtref : Inport  Port=2
  Enable : Inport  Port=3
  w_meas_Woodward : Inport  Port=4
  V_meas_Woodward : Inport  Port=5
  Woodward_Enable : Inport  Port=6
  Bus Creator1 : BusCreator
  Bus Creator3 : BusCreator  Inputs=3
  Bus Selector : BusSelector  OutputSignals=Vf_before,Vf_after
  Diesel Engine Speed & Voltage Control fast : Subsystem
  Synchronous Machine pu Fundamental : powerlib/Machines/Synchronous Machine pu Fundamental  PresetModel=22: 60Hz 460V 1075kVA 1800RPM  MechanicalLoad=Mechanical power Pm  ShowDetailedParameters=on  RotorType=Salient-pole  NominalParameters=[1.075e+006 460 60]  Stator=[0.01524 0.08 2.81 1.64]  Field=[0.004319 0.531]  Dampers2=[0.0652, 0.5134, 0.0287, 0.2553, 7.765e-3, 0.9167 ]  Dampers1=[0.2343 2.655 0.03365 0.2408]  Mechanical=[0.3222 0.01322 2]  PolePairs=2  InitialConditions="[ -99  0  0  0  0  0  0  0  0 ]"  SetSaturation=off  Saturation=[0.6404,0.7127,0.8441,0.9214,0.9956,1.082,1.19,1.316,1.457;0.7,0.7698,0.8872,0.9466,0.9969,1.046,1.1,1.151,1.201]  Units=per unit fundamental parameters  LoadFlowParameters=[1,0,0,0,0]  TsPowergui=0  TsBlock=-1  IterativeModel=Forward Euler  BusType=swing  Pref=0  Qref=0  Qmin=-inf  Qmax=inf  PLF=0  QLF=0
  A : PMIOPort  Port=1  Side=Right
  B : PMIOPort  Port=2  Side=Right
  C : PMIOPort  Port=3  Side=Right
  m : Outport
  Primary : Outport  Port=2
  wires:
  Vtref/1 -> Diesel Engine Speed & Voltage Control fast/2(Vtref)
  wref/1 -> Diesel Engine Speed & Voltage Control fast/1(wref)
  Diesel Engine Speed & Voltage Control fast/2(Vf) -> Synchronous Machine pu Fundamental/2, Bus Creator3/1  "vf"
  Diesel Engine Speed & Voltage Control fast/1(Pm) -> Synchronous Machine pu Fundamental/1, Bus Creator1/1  "Pm"
  Enable/1 -> Diesel Engine Speed & Voltage Control fast/3(Generator Enable)
  Synchronous Machine pu Fundamental/1 -> m/1, Diesel Engine Speed & Voltage Control fast/4(m)
  w_meas_Woodward/1 -> Diesel Engine Speed & Voltage Control fast/5(w_meas_Wood)
  V_meas_Woodward/1 -> Diesel Engine Speed & Voltage Control fast/6(V_meas_Wood)
  Diesel Engine Speed & Voltage Control fast/3(Vt) -> Bus Creator1/3  "vt"
  Diesel Engine Speed & Voltage Control fast/4(w) -> Bus Creator1/4  "w"
  Bus Creator1/1 -> Primary/1
  Diesel Engine Speed & Voltage Control fast/5(Misc) -> Bus Selector/1
  Bus Selector/1 -> Bus Creator3/2  "<Vf_before>"
  Bus Selector/2 -> Bus Creator3/3  "<Vf_after>"
  Bus Creator3/1 -> Bus Creator1/2  "Vf"
  Woodward_Enable/1 -> Diesel Engine Speed & Voltage Control fast/7(Woodward Enable)
  connections:
  C/RConn1 -- Synchronous Machine pu Fundamental/RConn3
  B/RConn1 -- Synchronous Machine pu Fundamental/RConn2
  A/RConn1 -- Synchronous Machine pu Fundamental/RConn1

== system MODEL_FULL_SYSTEM_MUTUAL/SM_Master/Generator_09222015/GenSet_1MVA_09082015/Interface between Woodward Controller and simated generator ==
  note: Note: This may need a different scaling because it is the reference signal.
      | Reference has to be between 0.95 and 1.05 pu in order to be in tolerance.
  Woodward for wref : Inport
  Woodward for Vref : Inport  Port=2
  Add2 : Sum
  Add3 : Sum
  Gain2 : Gain
  Gain3 : Gain
  Mux1 : Mux  Inputs=2
  Vref_set : Constant  Value=0
  wref_set : Constant  Value=0
  wref,Vref : Outport
  wires:
  Gain2/1 -> Add2/1  "bias"
  Add2/1 -> Mux1/1
  wref_set/1 -> Add2/2
  Gain3/1 -> Add3/1  "bias"
  Vref_set/1 -> Add3/2
  Add3/1 -> Mux1/2
  Woodward for wref/1 -> Gain2/1
  Mux1/1 -> wref,Vref/1  "hardware"
  Woodward for Vref/1 -> Gain3/1

== system MODEL_FULL_SYSTEM_MUTUAL/SM_Master/Generator_09222015/GenSet_1MVA_09082015/Simulated Generator Controller 900 kW ==
  Pref : Inport
  Qref : Inport  Port=2
  mode : Inport  Port=3
  set_vtref : Inport  Port=4
  set_wref : Inport  Port=5
  gen_m : Inport  Port=6
  Bus Selector1 : BusSelector  OutputSignals="Output active power   Peo (pu),Output reactive power  Qeo (pu)"
  Multiport Switch : MultiPortSwitch  zeroidx=off
  Mux1 : Mux  Inputs=2
  Mux2 : Mux  Inputs=2
  Mux3 : Mux  Inputs=2
  PQ control : Subsystem
  PV control : Subsystem
  "wref, Vref" : Outport
  wires:
  Bus Selector1/1 -> PQ control/2(P (pu)), PV control/2(P (pu))  "<Output active power   Peo (pu)>"
  gen_m/1 -> Bus Selector1/1
  PQ control/1(w_ref (pu)) -> Mux1/1
  PQ control/2(V_ref (pu)) -> Mux1/2
  PV control/1(w_ref (pu)) -> Mux2/1
  set_vtref/1 -> Mux2/2, Mux3/2
  Mux1/1 -> Multiport Switch/2
  Mux2/1 -> Multiport Switch/3
  Mux3/1 -> Multiport Switch/4
  Pref/1 -> PQ control/1(P_ref (pu)), PV control/1(P_ref (pu))
  Bus Selector1/2 -> PQ control/4(Q (pu))  "<Output reactive power  Qeo (pu)>"
  set_wref/1 -> Mux3/1
  Qref/1 -> PQ control/3(Q_ref (pu))
  mode/1 -> Multiport Switch/1
  Multiport Switch/1 -> "wref, Vref"/1

== system MODEL_FULL_SYSTEM_MUTUAL/SM_Master/Generator_09222015/GenSet_1MVA_09082015/StabilityL ==
  Constant Load : powerlib/Elements/Three-Phase Parallel RLC Load  LConnTagsString=A|B|C  Configuration=Y (grounded)  NominalVoltage=v  NominalFrequency=60  ActivePower=kVA*1E3*pf  InductivePower=kVA*1E3*sqrt(1-pf^2)  CapacitivePower=0  Measurements=None  LoadType=constant Z
  A : PMIOPort  Port=1  Side=Left
  B : PMIOPort  Port=2  Side=Left
  C : PMIOPort  Port=3  Side=Left
  connections:
  A/RConn1 -- Constant Load/LConn1
  B/RConn1 -- Constant Load/LConn2
  C/RConn1 -- Constant Load/LConn3

== system MODEL_FULL_SYSTEM_MUTUAL/SM_Master/Generator_09222015/GenSet_4MVA_09212015/4MVA Generator with  Primary Controllers1 ==
  wref : Inport
  Vtref : Inport  Port=2
  Enable : Inport  Port=3
  w_meas_Woodward : Inport  Port=4
  V_meas_Woodward : Inport  Port=5
  Woodward_Enable : Inport  Port=6
  Bus Creator1 : BusCreator
  Bus Creator3 : BusCreator  Inputs=3
  Bus Selector : BusSelector  OutputSignals=Vf_before,Vf_after
  Diesel Engine Speed & Voltage Control fast : Subsystem
  Synchronous Machine pu Fundamental : powerlib/Machines/Synchronous Machine pu Fundamental  PresetModel=No  MechanicalLoad=Mechanical power Pm  ShowDetailedParameters=on  RotorType=Salient-pole  NominalParameters=[4e+006 13800 60]  Stator=[0.008979 0.05 2.35 1.72]  Field=[0.00206 0.511]  Dampers2=[0.0652, 0.5134, 0.0287, 0.2553, 7.765e-3, 0.9167 ]  Dampers1=[0.2826 3.738 0.02545 0.2392]  Mechanical=[0.3468 0.009238 2]  PolePairs=2  InitialConditions="[ -99  0  0  0  0  0  0  0  0 ]"  SetSaturation=off  Saturation=[0.6404,0.7127,0.8441,0.9214,0.9956,1.082,1.19,1.316,1.457;0.7,0.7698,0.8872,0.9466,0.9969,1.046,1.1,1.151,1.201]  Units=per unit fundamental parameters  LoadFlowParameters=[1,0,0,0,0]  TsPowergui=0  TsBlock=-1  IterativeModel=Forward Euler  BusType=swing  Pref=0  Qref=0  Qmin=-inf  Qmax=inf  PLF=0  QLF=0
  A : PMIOPort  Port=1  Side=Right
  B : PMIOPort  Port=2  Side=Right
  C : PMIOPort  Port=3  Side=Right
  m : Outport
  Primary : Outport  Port=2
  wires:
  Woodward_Enable/1 -> Diesel Engine Speed & Voltage Control fast/7(Woodward Enable)
  Bus Creator3/1 -> Bus Creator1/2  "Vf"
  Bus Selector/2 -> Bus Creator3/3  "<Vf_after>"
  Bus Selector/1 -> Bus Creator3/2  "<Vf_before>"
  Diesel Engine Speed & Voltage Control fast/5(Misc) -> Bus Selector/1
  Bus Creator1/1 -> Primary/1
  Diesel Engine Speed & Voltage Control fast/4(w) -> Bus Creator1/4  "w"
  Diesel Engine Speed & Voltage Control fast/3(Vt) -> Bus Creator1/3  "vt"
  V_meas_Woodward/1 -> Diesel Engine Speed & Voltage Control fast/6(V_meas_Wood)
  w_meas_Woodward/1 -> Diesel Engine Speed & Voltage Control fast/5(w_meas_Wood)
  Synchronous Machine pu Fundamental/1 -> Diesel Engine Speed & Voltage Control fast/4(m), m/1
  Enable/1 -> Diesel Engine Speed & Voltage Control fast/3(Generator Enable)
  Diesel Engine Speed & Voltage Control fast/1(Pm) -> Bus Creator1/1, Synchronous Machine pu Fundamental/1  "Pm"
  Diesel Engine Speed & Voltage Control fast/2(Vf) -> Bus Creator3/1, Synchronous Machine pu Fundamental/2  "vf"
  wref/1 -> Diesel Engine Speed & Voltage Control fast/1(wref)
  Vtref/1 -> Diesel Engine Speed & Voltage Control fast/2(Vtref)
  connections:
  A/RConn1 -- Synchronous Machine pu Fundamental/RConn1
  B/RConn1 -- Synchronous Machine pu Fundamental/RConn2
  C/RConn1 -- Synchronous Machine pu Fundamental/RConn3

== system MODEL_FULL_SYSTEM_MUTUAL/SM_Master/Generator_09222015/GenSet_4MVA_09212015/Interface between Woodward Controller and simated generator ==
  note: Note: This may need a different scaling because it is the reference signal.
      | Reference has to be between 0.95 and 1.05 pu in order to be in tolerance.
  Woodward for wref : Inport
  Woodward for Vref : Inport  Port=2
  Add2 : Sum
  Add3 : Sum
  Gain2 : Gain
  Gain3 : Gain
  Mux1 : Mux  Inputs=2
  Vref_set : Constant  Value=0
  wref_set : Constant  Value=0
  wref,Vref : Outport
  wires:
  Gain2/1 -> Add2/1  "bias"
  Add2/1 -> Mux1/1
  wref_set/1 -> Add2/2
  Gain3/1 -> Add3/1  "bias"
  Vref_set/1 -> Add3/2
  Add3/1 -> Mux1/2
  Woodward for wref/1 -> Gain2/1
  Mux1/1 -> wref,Vref/1  "hardware"
  Woodward for Vref/1 -> Gain3/1

== system MODEL_FULL_SYSTEM_MUTUAL/SM_Master/Generator_09222015/GenSet_4MVA_09212015/Simulated Generator Controller 3.5 MW ==
  Pref : Inport
  Qref : Inport  Port=2
  mode : Inport  Port=3
  set_vtref : Inport  Port=4
  set_wref : Inport  Port=5
  gen_m : Inport  Port=6
  Bus Selector1 : BusSelector  OutputSignals="Output active power   Peo (pu),Output reactive power  Qeo (pu)"
  Multiport Switch : MultiPortSwitch  zeroidx=off
  Mux1 : Mux  Inputs=2
  Mux2 : Mux  Inputs=2
  Mux3 : Mux  Inputs=2
  PQ control : Subsystem
  PV control : Subsystem
  "wref, Vref" : Outport
  wires:
  Bus Selector1/1 -> PQ control/2(P (pu)), PV control/2(P (pu))  "<Output active power   Peo (pu)>"
  gen_m/1 -> Bus Selector1/1
  PQ control/1(w_ref (pu)) -> Mux1/1
  PQ control/2(V_ref (pu)) -> Mux1/2
  PV control/1(w_ref (pu)) -> Mux2/1
  set_vtref/1 -> Mux2/2, Mux3/2
  Mux1/1 -> Multiport Switch/2
  Mux2/1 -> Multiport Switch/3
  Mux3/1 -> Multiport Switch/4
  Pref/1 -> PQ control/1(P_ref (pu)), PV control/1(P_ref (pu))
  Bus Selector1/2 -> PQ control/4(Q (pu))  "<Output reactive power  Qeo (pu)>"
  set_wref/1 -> Mux3/1
  Qref/1 -> PQ control/3(Q_ref (pu))
  mode/1 -> Multiport Switch/1
  Multiport Switch/1 -> "wref, Vref"/1

== system MODEL_FULL_SYSTEM_MUTUAL/SM_Master/Generator_09222015/GenSet_4MVA_09212015/StabilityL ==
  Constant Load : powerlib/Elements/Three-Phase Parallel RLC Load  LConnTagsString=A|B|C  Configuration=Y (grounded)  NominalVoltage=v  NominalFrequency=60  ActivePower=kVA*1E3*pf  InductivePower=kVA*1E3*sqrt(1-pf^2)  CapacitivePower=0  Measurements=None  LoadType=constant Z
  A : PMIOPort  Port=1  Side=Left
  B : PMIOPort  Port=2  Side=Left
  C : PMIOPort  Port=3  Side=Left
  connections:
  A/RConn1 -- Constant Load/LConn1
  B/RConn1 -- Constant Load/LConn2
  C/RConn1 -- Constant Load/LConn3
